simulink model "parallel_prediction_and_cost_function_6phase"  (R2022a)
settings: Solver=FixedStepDiscrete  StartTime=0.0  StopTime=10.0  RelTol=1e-3
undefined symbols (not defined in the file): f_c, L_d, L_q, L_x, L_y, p, psi_pm, R_ph
libraries: hdlsllib x5
(part 3 of 3)

== system parallel_prediction_and_cost_function_6phase/Prediction_and_cost_function/Subsystem/Subsystem4 ==
  id_ref : Inport
  iq_ref : Inport  Port=2
  SampleTime_div_Ld : Inport  Port=3
  SampleTime_div_Lq : Inport  Port=4
  SampleTime_div_Lx : Inport  Port=5
  SampleTime_div_Ly : Inport  Port=6
  d_phase_voltage_per_switching_state : Inport  Port=7
  q_phase_voltage_per_switching_state : Inport  Port=8
  x_phase_voltage_per_switching_state : Inport  Port=9
  y_phase_voltage_per_switching_state : Inport  Port=10
  ix_ref : Inport  Port=11
  id_k : Inport  Port=12
  iq_k : Inport  Port=13
  ix_k : Inport  Port=14
  iy_k : Inport  Port=15
  psiPM : Inport  Port=16
  Lq : Inport  Port=17
  iy_ref : Inport  Port=18
  Ld : Inport  Port=19
  Rs : Inport  Port=20
  omega_el : Inport  Port=21
  Add{,1,3..4} (4 alike) : Sum  OutDataTypeStr=single
  Add2 : Sum
  Product{1..2,4..11} (10 alike) : Product  OutDataTypeStr=single
  Product3 : Product  Inputs=3  OutDataTypeStr=single
  Square{1..4} (4 alike) : Math  Operator=square  SignedPower=on  RndMeth=Zero
  Subtract : Sum  Inputs=+-+  OutDataTypeStr=single
  Subtract1 : Sum  Inputs=+--  OutDataTypeStr=single
  Subtract2 : Sum  Inputs=+-  OutDataTypeStr=single
  Subtract3 : Sum  Inputs=+-  OutDataTypeStr=single
  Subtract{4..7} (4 alike) : Sum  Inputs=+-
  Sum of Elements : Sum  Inputs=++++
  J : Outport
  wires:
  Add1/1 -> Subtract5/2
  q_phase_voltage_per_switching_state/1 -> Subtract1/1
  ix_ref/1 -> Subtract6/1
  omega_el/1 -> Product3/1, Product6/1
  Product5/1 -> Subtract1/2
  iq_k/1 -> Product3/3, Add1/2, Product5/1
  iy_k/1 -> Add4/2, Product11/1
  Add2/1 -> Product6/2
  Lq/1 -> Product3/2
  Add4/1 -> Subtract7/2
  Subtract2/1 -> Product8/2
  SampleTime_div_Ly/1 -> Product10/1
  Rs/1 -> Product9/2, Product2/2, Product5/2, Product11/2
  Product9/1 -> Subtract2/2
  Product8/1 -> Add3/1
  Product7/1 -> Add2/2
  id_k/1 -> Add/2, Product2/1, Product7/1
  x_phase_voltage_per_switching_state/1 -> Subtract2/1
  Add3/1 -> Subtract6/2
  Add/1 -> Subtract4/2
  Product11/1 -> Subtract3/2
  Product6/1 -> Subtract1/3
  Subtract1/1 -> Product4/2
  Product1/1 -> Add/1
  Product10/1 -> Add4/1
  Product4/1 -> Add1/1
  SampleTime_div_Ld/1 -> Product1/1
  y_phase_voltage_per_switching_state/1 -> Subtract3/1
  Product2/1 -> Subtract/2
  Subtract5/1 -> Square1/1
  Product3/1 -> Subtract/3
  SampleTime_div_Lq/1 -> Product4/1
  Subtract/1 -> Product1/2
  Subtract3/1 -> Product10/2
  Sum of Elements/1 -> J/1  "J"
  psiPM/1 -> Add2/1
  id_ref/1 -> Subtract4/1
  Subtract6/1 -> Square2/1
  Ld/1 -> Product7/2
  iy_ref/1 -> Subtract7/1
  ix_k/1 -> Add3/2, Product9/1
  Subtract4/1 -> Square4/1
  Subtract7/1 -> Square3/1
  iq_ref/1 -> Subtract5/1
  SampleTime_div_Lx/1 -> Product8/1
  d_phase_voltage_per_switching_state/1 -> Subtract/1
  Square3/1 -> Sum of Elements/4
  Square2/1 -> Sum of Elements/3
  Square1/1 -> Sum of Elements/2
  Square4/1 -> Sum of Elements/1

== system parallel_prediction_and_cost_function_6phase/Prediction_and_cost_function/Subsystem/Subsystem5 ==
  id_ref : Inport
  iq_ref : Inport  Port=2
  SampleTime_div_Ld : Inport  Port=3
  SampleTime_div_Lq : Inport  Port=4
  SampleTime_div_Lx : Inport  Port=5
  SampleTime_div_Ly : Inport  Port=6
  d_phase_voltage_per_switching_state : Inport  Port=7
  q_phase_voltage_per_switching_state : Inport  Port=8
  x_phase_voltage_per_switching_state : Inport  Port=9
  y_phase_voltage_per_switching_state : Inport  Port=10
  ix_ref : Inport  Port=11
  id_k : Inport  Port=12
  iq_k : Inport  Port=13
  ix_k : Inport  Port=14
  iy_k : Inport  Port=15
  psiPM : Inport  Port=16
  Lq : Inport  Port=17
  iy_ref : Inport  Port=18
  Ld : Inport  Port=19
  Rs : Inport  Port=20
  omega_el : Inport  Port=21
  Add{,1,3..4} (4 alike) : Sum  OutDataTypeStr=single
  Add2 : Sum
  Product{1..2,4..11} (10 alike) : Product  OutDataTypeStr=single
  Product3 : Product  Inputs=3  OutDataTypeStr=single
  Square{1..4} (4 alike) : Math  Operator=square  SignedPower=on  RndMeth=Zero
  Subtract : Sum  Inputs=+-+  OutDataTypeStr=single
  Subtract1 : Sum  Inputs=+--  OutDataTypeStr=single
  Subtract2 : Sum  Inputs=+-  OutDataTypeStr=single
  Subtract3 : Sum  Inputs=+-  OutDataTypeStr=single
  Subtract{4..7} (4 alike) : Sum  Inputs=+-
  Sum of Elements : Sum  Inputs=++++
  J : Outport
  wires:
  Add1/1 -> Subtract5/2
  q_phase_voltage_per_switching_state/1 -> Subtract1/1
  ix_ref/1 -> Subtract6/1
  omega_el/1 -> Product3/1, Product6/1
  Product5/1 -> Subtract1/2
  iq_k/1 -> Product3/3, Add1/2, Product5/1
  iy_k/1 -> Add4/2, Product11/1
  Add2/1 -> Product6/2
  Lq/1 -> Product3/2
  Add4/1 -> Subtract7/2
  Subtract2/1 -> Product8/2
  SampleTime_div_Ly/1 -> Product10/1
  Rs/1 -> Product9/2, Product2/2, Product5/2, Product11/2
  Product9/1 -> Subtract2/2
  Product8/1 -> Add3/1
  Product7/1 -> Add2/2
  id_k/1 -> Add/2, Product2/1, Product7/1
  x_phase_voltage_per_switching_state/1 -> Subtract2/1
  Add3/1 -> Subtract6/2
  Add/1 -> Subtract4/2
  Product11/1 -> Subtract3/2
  Product6/1 -> Subtract1/3
  Subtract1/1 -> Product4/2
  Product1/1 -> Add/1
  Product10/1 -> Add4/1
  Product4/1 -> Add1/1
  SampleTime_div_Ld/1 -> Product1/1
  y_phase_voltage_per_switching_state/1 -> Subtract3/1
  Product2/1 -> Subtract/2
  Subtract5/1 -> Square1/1
  Product3/1 -> Subtract/3
  SampleTime_div_Lq/1 -> Product4/1
  Subtract/1 -> Product1/2
  Subtract3/1 -> Product10/2
  Sum of Elements/1 -> J/1  "J"
  psiPM/1 -> Add2/1
  id_ref/1 -> Subtract4/1
  Subtract6/1 -> Square2/1
  Ld/1 -> Product7/2
  iy_ref/1 -> Subtract7/1
  ix_k/1 -> Add3/2, Product9/1
  Subtract4/1 -> Square4/1
  Subtract7/1 -> Square3/1
  iq_ref/1 -> Subtract5/1
  SampleTime_div_Lx/1 -> Product8/1
  d_phase_voltage_per_switching_state/1 -> Subtract/1
  Square3/1 -> Sum of Elements/4
  Square2/1 -> Sum of Elements/3
  Square1/1 -> Sum of Elements/2
  Square4/1 -> Sum of Elements/1

== system parallel_prediction_and_cost_function_6phase/Prediction_and_cost_function/Subsystem/Subsystem6 ==
  id_ref : Inport
  iq_ref : Inport  Port=2
  SampleTime_div_Ld : Inport  Port=3
  SampleTime_div_Lq : Inport  Port=4
  SampleTime_div_Lx : Inport  Port=5
  SampleTime_div_Ly : Inport  Port=6
  d_phase_voltage_per_switching_state : Inport  Port=7
  q_phase_voltage_per_switching_state : Inport  Port=8
  x_phase_voltage_per_switching_state : Inport  Port=9
  y_phase_voltage_per_switching_state : Inport  Port=10
  ix_ref : Inport  Port=11
  id_k : Inport  Port=12
  iq_k : Inport  Port=13
  ix_k : Inport  Port=14
  iy_k : Inport  Port=15
  psiPM : Inport  Port=16
  Lq : Inport  Port=17
  iy_ref : Inport  Port=18
  Ld : Inport  Port=19
  Rs : Inport  Port=20
  omega_el : Inport  Port=21
  Add{,1,3..4} (4 alike) : Sum  OutDataTypeStr=single
  Add2 : Sum
  Product{1..2,4..11} (10 alike) : Product  OutDataTypeStr=single
  Product3 : Product  Inputs=3  OutDataTypeStr=single
  Square{1..4} (4 alike) : Math  Operator=square  SignedPower=on  RndMeth=Zero
  Subtract : Sum  Inputs=+-+  OutDataTypeStr=single
  Subtract1 : Sum  Inputs=+--  OutDataTypeStr=single
  Subtract2 : Sum  Inputs=+-  OutDataTypeStr=single
  Subtract3 : Sum  Inputs=+-  OutDataTypeStr=single
  Subtract{4..7} (4 alike) : Sum  Inputs=+-
  Sum of Elements : Sum  Inputs=++++
  J : Outport
  wires:
  Add1/1 -> Subtract5/2
  q_phase_voltage_per_switching_state/1 -> Subtract1/1
  ix_ref/1 -> Subtract6/1
  omega_el/1 -> Product3/1, Product6/1
  Product5/1 -> Subtract1/2
  iq_k/1 -> Product3/3, Add1/2, Product5/1
  iy_k/1 -> Add4/2, Product11/1
  Add2/1 -> Product6/2
  Lq/1 -> Product3/2
  Add4/1 -> Subtract7/2
  Subtract2/1 -> Product8/2
  SampleTime_div_Ly/1 -> Product10/1
  Rs/1 -> Product9/2, Product2/2, Product5/2, Product11/2
  Product9/1 -> Subtract2/2
  Product8/1 -> Add3/1
  Product7/1 -> Add2/2
  id_k/1 -> Add/2, Product2/1, Product7/1
  x_phase_voltage_per_switching_state/1 -> Subtract2/1
  Add3/1 -> Subtract6/2
  Add/1 -> Subtract4/2
  Product11/1 -> Subtract3/2
  Product6/1 -> Subtract1/3
  Subtract1/1 -> Product4/2
  Product1/1 -> Add/1
  Product10/1 -> Add4/1
  Product4/1 -> Add1/1
  SampleTime_div_Ld/1 -> Product1/1
  y_phase_voltage_per_switching_state/1 -> Subtract3/1
  Product2/1 -> Subtract/2
  Subtract5/1 -> Square1/1
  Product3/1 -> Subtract/3
  SampleTime_div_Lq/1 -> Product4/1
  Subtract/1 -> Product1/2
  Subtract3/1 -> Product10/2
  Sum of Elements/1 -> J/1  "J"
  psiPM/1 -> Add2/1
  id_ref/1 -> Subtract4/1
  Subtract6/1 -> Square2/1
  Ld/1 -> Product7/2
  iy_ref/1 -> Subtract7/1
  ix_k/1 -> Add3/2, Product9/1
  Subtract4/1 -> Square4/1
  Subtract7/1 -> Square3/1
  iq_ref/1 -> Subtract5/1
  SampleTime_div_Lx/1 -> Product8/1
  d_phase_voltage_per_switching_state/1 -> Subtract/1
  Square3/1 -> Sum of Elements/4
  Square2/1 -> Sum of Elements/3
  Square1/1 -> Sum of Elements/2
  Square4/1 -> Sum of Elements/1

== system parallel_prediction_and_cost_function_6phase/Prediction_and_cost_function/Subsystem/Subsystem7 ==
  id_ref : Inport
  iq_ref : Inport  Port=2
  SampleTime_div_Ld : Inport  Port=3
  SampleTime_div_Lq : Inport  Port=4
  SampleTime_div_Lx : Inport  Port=5
  SampleTime_div_Ly : Inport  Port=6
  d_phase_voltage_per_switching_state : Inport  Port=7
  q_phase_voltage_per_switching_state : Inport  Port=8
  x_phase_voltage_per_switching_state : Inport  Port=9
  y_phase_voltage_per_switching_state : Inport  Port=10
  ix_ref : Inport  Port=11
  id_k : Inport  Port=12
  iq_k : Inport  Port=13
  ix_k : Inport  Port=14
  iy_k : Inport  Port=15
  psiPM : Inport  Port=16
  Lq : Inport  Port=17
  iy_ref : Inport  Port=18
  Ld : Inport  Port=19
  Rs : Inport  Port=20
  omega_el : Inport  Port=21
  Add{,1,3..4} (4 alike) : Sum  OutDataTypeStr=single
  Add2 : Sum
  Product{1..2,4..11} (10 alike) : Product  OutDataTypeStr=single
  Product3 : Product  Inputs=3  OutDataTypeStr=single
  Square{1..4} (4 alike) : Math  Operator=square  SignedPower=on  RndMeth=Zero
  Subtract : Sum  Inputs=+-+  OutDataTypeStr=single
  Subtract1 : Sum  Inputs=+--  OutDataTypeStr=single
  Subtract2 : Sum  Inputs=+-  OutDataTypeStr=single
  Subtract3 : Sum  Inputs=+-  OutDataTypeStr=single
  Subtract{4..7} (4 alike) : Sum  Inputs=+-
  Sum of Elements : Sum  Inputs=++++
  J : Outport
  wires:
  Add1/1 -> Subtract5/2
  q_phase_voltage_per_switching_state/1 -> Subtract1/1
  ix_ref/1 -> Subtract6/1
  omega_el/1 -> Product3/1, Product6/1
  Product5/1 -> Subtract1/2
  iq_k/1 -> Product3/3, Add1/2, Product5/1
  iy_k/1 -> Add4/2, Product11/1
  Add2/1 -> Product6/2
  Lq/1 -> Product3/2
  Add4/1 -> Subtract7/2
  Subtract2/1 -> Product8/2
  SampleTime_div_Ly/1 -> Product10/1
  Rs/1 -> Product9/2, Product2/2, Product5/2, Product11/2
  Product9/1 -> Subtract2/2
  Product8/1 -> Add3/1
  Product7/1 -> Add2/2
  id_k/1 -> Add/2, Product2/1, Product7/1
  x_phase_voltage_per_switching_state/1 -> Subtract2/1
  Add3/1 -> Subtract6/2
  Add/1 -> Subtract4/2
  Product11/1 -> Subtract3/2
  Product6/1 -> Subtract1/3
  Subtract1/1 -> Product4/2
  Product1/1 -> Add/1
  Product10/1 -> Add4/1
  Product4/1 -> Add1/1
  SampleTime_div_Ld/1 -> Product1/1
  y_phase_voltage_per_switching_state/1 -> Subtract3/1
  Product2/1 -> Subtract/2
  Subtract5/1 -> Square1/1
  Product3/1 -> Subtract/3
  SampleTime_div_Lq/1 -> Product4/1
  Subtract/1 -> Product1/2
  Subtract3/1 -> Product10/2
  Sum of Elements/1 -> J/1  "J"
  psiPM/1 -> Add2/1
  id_ref/1 -> Subtract4/1
  Subtract6/1 -> Square2/1
  Ld/1 -> Product7/2
  iy_ref/1 -> Subtract7/1
  ix_k/1 -> Add3/2, Product9/1
  Subtract4/1 -> Square4/1
  Subtract7/1 -> Square3/1
  iq_ref/1 -> Subtract5/1
  SampleTime_div_Lx/1 -> Product8/1
  d_phase_voltage_per_switching_state/1 -> Subtract/1
  Square3/1 -> Sum of Elements/4
  Square2/1 -> Sum of Elements/3
  Square1/1 -> Sum of Elements/2
  Square4/1 -> Sum of Elements/1

== system parallel_prediction_and_cost_function_6phase/Prediction_and_cost_function/Subsystem/Subsystem8 ==
  id_ref : Inport
  iq_ref : Inport  Port=2
  SampleTime_div_Ld : Inport  Port=3
  SampleTime_div_Lq : Inport  Port=4
  SampleTime_div_Lx : Inport  Port=5
  SampleTime_div_Ly : Inport  Port=6
  d_phase_voltage_per_switching_state : Inport  Port=7
  q_phase_voltage_per_switching_state : Inport  Port=8
  x_phase_voltage_per_switching_state : Inport  Port=9
  y_phase_voltage_per_switching_state : Inport  Port=10
  ix_ref : Inport  Port=11
  id_k : Inport  Port=12
  iq_k : Inport  Port=13
  ix_k : Inport  Port=14
  iy_k : Inport  Port=15
  psiPM : Inport  Port=16
  Lq : Inport  Port=17
  iy_ref : Inport  Port=18
  Ld : Inport  Port=19
  Rs : Inport  Port=20
  omega_el : Inport  Port=21
  Add{,1,3..4} (4 alike) : Sum  OutDataTypeStr=single
  Add2 : Sum
  Product{1..2,4..11} (10 alike) : Product  OutDataTypeStr=single
  Product3 : Product  Inputs=3  OutDataTypeStr=single
  Square{1..4} (4 alike) : Math  Operator=square  SignedPower=on  RndMeth=Zero
  Subtract : Sum  Inputs=+-+  OutDataTypeStr=single
  Subtract1 : Sum  Inputs=+--  OutDataTypeStr=single
  Subtract2 : Sum  Inputs=+-  OutDataTypeStr=single
  Subtract3 : Sum  Inputs=+-  OutDataTypeStr=single
  Subtract{4..7} (4 alike) : Sum  Inputs=+-
  Sum of Elements : Sum  Inputs=++++
  J : Outport
  wires:
  Add1/1 -> Subtract5/2
  q_phase_voltage_per_switching_state/1 -> Subtract1/1
  ix_ref/1 -> Subtract6/1
  omega_el/1 -> Product3/1, Product6/1
  Product5/1 -> Subtract1/2
  iq_k/1 -> Product3/3, Add1/2, Product5/1
  iy_k/1 -> Add4/2, Product11/1
  Add2/1 -> Product6/2
  Lq/1 -> Product3/2
  Add4/1 -> Subtract7/2
  Subtract2/1 -> Product8/2
  SampleTime_div_Ly/1 -> Product10/1
  Rs/1 -> Product9/2, Product2/2, Product5/2, Product11/2
  Product9/1 -> Subtract2/2
  Product8/1 -> Add3/1
  Product7/1 -> Add2/2
  id_k/1 -> Add/2, Product2/1, Product7/1
  x_phase_voltage_per_switching_state/1 -> Subtract2/1
  Add3/1 -> Subtract6/2
  Add/1 -> Subtract4/2
  Product11/1 -> Subtract3/2
  Product6/1 -> Subtract1/3
  Subtract1/1 -> Product4/2
  Product1/1 -> Add/1
  Product10/1 -> Add4/1
  Product4/1 -> Add1/1
  SampleTime_div_Ld/1 -> Product1/1
  y_phase_voltage_per_switching_state/1 -> Subtract3/1
  Product2/1 -> Subtract/2
  Subtract5/1 -> Square1/1
  Product3/1 -> Subtract/3
  SampleTime_div_Lq/1 -> Product4/1
  Subtract/1 -> Product1/2
  Subtract3/1 -> Product10/2
  Sum of Elements/1 -> J/1  "J"
  psiPM/1 -> Add2/1
  id_ref/1 -> Subtract4/1
  Subtract6/1 -> Square2/1
  Ld/1 -> Product7/2
  iy_ref/1 -> Subtract7/1
  ix_k/1 -> Add3/2, Product9/1
  Subtract4/1 -> Square4/1
  Subtract7/1 -> Square3/1
  iq_ref/1 -> Subtract5/1
  SampleTime_div_Lx/1 -> Product8/1
  d_phase_voltage_per_switching_state/1 -> Subtract/1
  Square3/1 -> Sum of Elements/4
  Square2/1 -> Sum of Elements/3
  Square1/1 -> Sum of Elements/2
  Square4/1 -> Sum of Elements/1

== system parallel_prediction_and_cost_function_6phase/Prediction_and_cost_function/Subsystem/Subsystem9 ==
  id_ref : Inport
  iq_ref : Inport  Port=2
  SampleTime_div_Ld : Inport  Port=3
  SampleTime_div_Lq : Inport  Port=4
  SampleTime_div_Lx : Inport  Port=5
  SampleTime_div_Ly : Inport  Port=6
  d_phase_voltage_per_switching_state : Inport  Port=7
  q_phase_voltage_per_switching_state : Inport  Port=8
  x_phase_voltage_per_switching_state : Inport  Port=9
  y_phase_voltage_per_switching_state : Inport  Port=10
  ix_ref : Inport  Port=11
  id_k : Inport  Port=12
  iq_k : Inport  Port=13
  ix_k : Inport  Port=14
  iy_k : Inport  Port=15
  psiPM : Inport  Port=16
  Lq : Inport  Port=17
  iy_ref : Inport  Port=18
  Ld : Inport  Port=19
  Rs : Inport  Port=20
  omega_el : Inport  Port=21
  Add{,1,3..4} (4 alike) : Sum  OutDataTypeStr=single
  Add2 : Sum
  Product{1..2,4..11} (10 alike) : Product  OutDataTypeStr=single
  Product3 : Product  Inputs=3  OutDataTypeStr=single
  Square{1..4} (4 alike) : Math  Operator=square  SignedPower=on  RndMeth=Zero
  Subtract : Sum  Inputs=+-+  OutDataTypeStr=single
  Subtract1 : Sum  Inputs=+--  OutDataTypeStr=single
  Subtract2 : Sum  Inputs=+-  OutDataTypeStr=single
  Subtract3 : Sum  Inputs=+-  OutDataTypeStr=single
  Subtract{4..7} (4 alike) : Sum  Inputs=+-
  Sum of Elements : Sum  Inputs=++++
  J : Outport
  wires:
  Add1/1 -> Subtract5/2
  q_phase_voltage_per_switching_state/1 -> Subtract1/1
  ix_ref/1 -> Subtract6/1
  omega_el/1 -> Product3/1, Product6/1
  Product5/1 -> Subtract1/2
  iq_k/1 -> Product3/3, Add1/2, Product5/1
  iy_k/1 -> Add4/2, Product11/1
  Add2/1 -> Product6/2
  Lq/1 -> Product3/2
  Add4/1 -> Subtract7/2
  Subtract2/1 -> Product8/2
  SampleTime_div_Ly/1 -> Product10/1
  Rs/1 -> Product9/2, Product2/2, Product5/2, Product11/2
  Product9/1 -> Subtract2/2
  Product8/1 -> Add3/1
  Product7/1 -> Add2/2
  id_k/1 -> Add/2, Product2/1, Product7/1
  x_phase_voltage_per_switching_state/1 -> Subtract2/1
  Add3/1 -> Subtract6/2
  Add/1 -> Subtract4/2
  Product11/1 -> Subtract3/2
  Product6/1 -> Subtract1/3
  Subtract1/1 -> Product4/2
  Product1/1 -> Add/1
  Subtract7/1 -> Square3/1
  Product10/1 -> Add4/1
  Product4/1 -> Add1/1
  SampleTime_div_Ld/1 -> Product1/1
  y_phase_voltage_per_switching_state/1 -> Subtract3/1
  Product2/1 -> Subtract/2
  Subtract5/1 -> Square1/1
  Product3/1 -> Subtract/3
  SampleTime_div_Lq/1 -> Product4/1
  Subtract/1 -> Product1/2
  Subtract3/1 -> Product10/2
  Sum of Elements/1 -> J/1  "J"
  psiPM/1 -> Add2/1
  id_ref/1 -> Subtract4/1
  Subtract6/1 -> Square2/1
  Square2/1 -> Sum of Elements/3
  Ld/1 -> Product7/2
  iy_ref/1 -> Subtract7/1
  ix_k/1 -> Add3/2, Product9/1
  Subtract4/1 -> Square4/1
  Square3/1 -> Sum of Elements/4
  iq_ref/1 -> Subtract5/1
  SampleTime_div_Lx/1 -> Product8/1
  d_phase_voltage_per_switching_state/1 -> Subtract/1
  Square1/1 -> Sum of Elements/2
  Square4/1 -> Sum of Elements/1
